simulink model "SimX"  (Simulink 9.2)
settings: Solver=ode45  StartTime=0.0  StopTime=TqB+TqS  RelTol=1e-3  EnableMultiTasking=on
values from neighbouring files (symbols this model uses):
  Mf = Mtot - Mp_tot    [dimensionamento_exocet.m]    (also in dimensionamento_resultados.mat = 514.4)
  SRef = pi*DRef^2/4    (= 0.0962112750162)    [dimensionamento_exocet.m]    (also in dimensionamento_resultados.mat)
  VCd = [0    0.33 ... (first row only)    [dimensionamento_exocet.m]
undefined symbols (not defined in the file or in its folder): Ro, Vi, VProp, VSom
settings Model: Creator=Administrador  LastModifiedBy=carlberto-old
settings OptimizationCC: ExpressionDepthLimit=2147483647

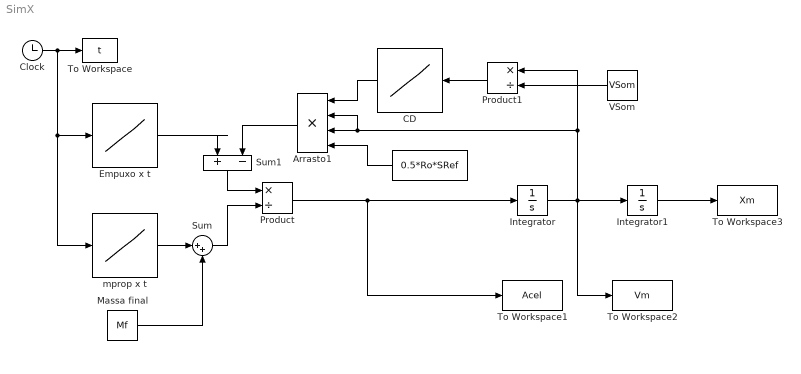
== system SimX ==
  " " : Constant  Value=0.5*Ro*SRef
  Arrasto1 : Product  Inputs=****
  CD : Lookup_n-D  NumberOfTableDimensions=1  BreakpointsForDimension1=VCd(:,1)  Table=VCd(:,2)  ExtrapMethod=Clip  RndMeth=Simplest  InputSameDT=on
  Clock : Clock
  Empuxo x t : Lookup_n-D  NumberOfTableDimensions=1  BreakpointsForDimension1=VProp(:,1)  Table=VProp(:,2)  ExtrapMethod=Clip  RndMeth=Simplest  InputSameDT=on
  Integrator : Integrator  InitialCondition=Vi
  Integrator1 : Integrator
  Massa final : Constant  Value=Mf
  Product : Product  Inputs=*/  RndMeth=Zero
  Product1 : Product  Inputs=*/  RndMeth=Zero
  Sum : Sum  Inputs=|++
  Sum1 : Sum  Inputs=|+-
  To Workspace : ToWorkspace  VariableName=t  SampleTime=-1
  To Workspace1 : ToWorkspace  VariableName=Acel  SampleTime=-1
  To Workspace2 : ToWorkspace  VariableName=Vm  SampleTime=-1
  To Workspace3 : ToWorkspace  VariableName=Xm  SampleTime=-1
  VSom : Constant  Value=VSom
  mprop x t : Lookup_n-D  NumberOfTableDimensions=1  BreakpointsForDimension1=VProp(:,1)  Table=VProp(:,3)  ExtrapMethod=Clip  RndMeth=Simplest  InputSameDT=on
  wires:
  Clock/1 -> To Workspace/1, Empuxo x t/1, mprop x t/1
  mprop x t/1 -> Sum/1
  Massa final/1 -> Sum/2
  Sum/1 -> Product/2
  Integrator/1 -> Integrator1/1, To Workspace2/1, Product1/1, Arrasto1/3, Arrasto1/2
  Integrator1/1 -> To Workspace3/1
  Product1/1 -> CD/1
  VSom/1 -> Product1/2
  Empuxo x t/1 -> Sum1/1
  Sum1/1 -> Product/1
  Product/1 -> Integrator/1, To Workspace1/1
  CD/1 -> Arrasto1/1
  " "/1 -> Arrasto1/4
  Arrasto1/1 -> Sum1/2
